simulink model "SimulinkModelP"  (R2019b)
settings: Solver=VariableStepAuto  StartTime=0.0  StopTime=50000  RelTol=1e-7
settings Model: Creator=Jad Yahya  LastModifiedBy=Jad Yahya

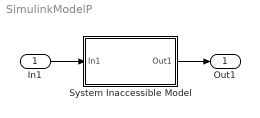
== system SimulinkModelP ==
  In1 : Inport
  System Inaccessible Model : Subsystem
  Out1 : Outport
  wires:
  In1/1 -> System Inaccessible Model/1(In1)
  System Inaccessible Model/1(Out1) -> Out1/1

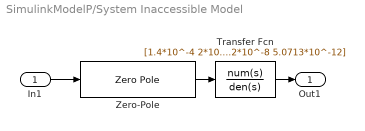
== system SimulinkModelP/System Inaccessible Model ==
  In1 : Inport
  Transfer Fcn : TransferFcn  Numerator=[1.4*10^-4 2*10^-7 7.56*10^-12]  Denominator=[1 3.68*10^-2 2.35752*10^-4 8.2*10^-8 5.0713*10^-12]
  Zero-Pole : ZeroPole  Zeros=[0.2353]  Poles=[ -0.2353]  Gain=[-1]
  Out1 : Outport
  wires:
  In1/1 -> Zero-Pole/1
  Zero-Pole/1 -> Transfer Fcn/1
  Transfer Fcn/1 -> Out1/1
